simulink model "controlSimulation"  (R2018a)
settings: Solver=VariableStepAuto  StartTime=0.0  StopTime=30  FixedStep=0.01  MaxStep=0.05  RelTol=1e-3  EnableMultiTasking=on
libraries: simulink x1
settings Model: Creator=kk  LastModifiedBy=kk
settings DataIOCC: LimitDataPoints=on  SaveFormat=Array  SaveOutput=off  SignalLogging=off  DSMLogging=off  SaveTime=off
settings OptimizationCC: LifeSpan=inf
settings DebuggingCC: SolverPrmCheckMsg=warning  SFUnexpectedBacktrackingDiag=warning  SFNoUnconditionalDefaultTransitionDiag=warning  SFExecutionAtInitializationDiag=none
settings HardwareCC: ProdBitPerPointer=32  ProdBitPerSizeT=32  ProdBitPerPtrDiffT=32  ProdLargestAtomicFloat=None  ProdIntDivRoundTo=Undefined  ProdEndianess=Unspecified  ProdWordSize=32  ProdHWDeviceType=32-bit Generic
settings ModelReferenceCC: PropagateSignalLabelsOutOfModel=off
settings CodeAppCC: StateflowObjectComments=on
settings GRTTargetCC: TargetLangStandard=C89/C90 (ANSI)  GeneratePreprocessorConditionals=Disable all
settings ConfigComp: CovMetricSettings=dw  CovHtmlReporting=on  CovSaveCumulativeToWorkspaceVar=on  CovSaveSingleToWorkspaceVar=on  CovExternalEMLEnable=off  CovSFcnEnable=off

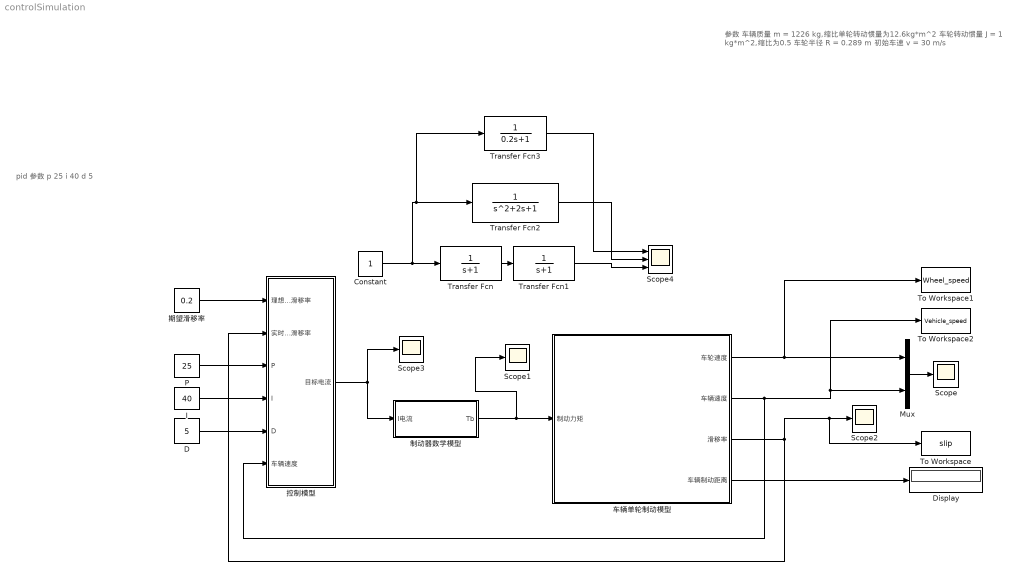
== system controlSimulation ==
  note: pid 参数
      | p 25
      | i 40
      | d 5
  note: 参数
      | 车辆质量 m = 1226 kg,缩比单轮转动惯量为12.6kg*m^2
      | 车轮转动惯量 J = 1 kg*m^2,缩比为0.5
      | 车轮半径 R = 0.289 m
      | 初始车速 v = 30 m/s
  Constant : Constant
  D : Constant  Value=5
  Display : Display
  I : Constant  Value=40
  Mux : Mux  Inputs=2
  P : Constant  Value=25
  Scope{,1..3} (4 alike) : Scope
  Scope4 : Scope  NumInputPorts=3
  To Workspace : ToWorkspace  VariableName=slip  SaveFormat=Timeseries  SampleTime=-1
  To Workspace1 : ToWorkspace  VariableName=Wheel_speed  SaveFormat=Timeseries  SampleTime=-1
  To Workspace2 : ToWorkspace  VariableName=Vehicle_speed  SaveFormat=Timeseries  SampleTime=-1
  Transfer Fcn : TransferFcn  Numerator=1  Denominator=[1 1]
  Transfer Fcn1 : TransferFcn  Numerator=1  Denominator=[1 1]
  Transfer Fcn2 : TransferFcn  Numerator=1
  Transfer Fcn3 : TransferFcn  Numerator=1  Denominator=[0.2 1]
  制动器数学模型 : Subsystem
  控制模型 : Subsystem
  期望滑移率 : Constant  Value=0.2
  车辆单轮制动模型 : Subsystem  mask{v=30, r=0.289, I=0.98/2, m=306.5/2, g=9.8, att=1}
      mask prompts: v "InitialVelocity(v  m/s)"; r "RollingRadius"; I "inertia of a wheel"; m "1/4 Vehicle weight"; g "GravityAcceleration"; att "Attachment condition"
      mask TypeOptions att: 1 | 2 | 3
      mask DialogControl Control2 Prompt: high 1 mediam 2 low 3
  wires:
  期望滑移率/1 -> 控制模型/1(理想滑移率)
  车辆单轮制动模型/3(滑移率) -> To Workspace/1, Scope2/1, 控制模型/2(实时滑移率)
  车辆单轮制动模型/1(车轮速度) -> To Workspace1/1, Mux/1
  Mux/1 -> Scope/1
  P/1 -> 控制模型/3(P)
  I/1 -> 控制模型/4(I)
  D/1 -> 控制模型/5(D)
  车辆单轮制动模型/4(车辆制动距离) -> Display/1
  制动器数学模型/1(Tb) -> Scope1/1, 车辆单轮制动模型/1(制动力矩)
  控制模型/1(目标电流) -> Scope3/1, 制动器数学模型/1(I电流)
  车辆单轮制动模型/2(车辆速度) -> To Workspace2/1, Mux/2, 控制模型/6(车辆速度)
  Constant/1 -> Transfer Fcn3/1, Transfer Fcn2/1, Transfer Fcn/1
  Transfer Fcn/1 -> Transfer Fcn1/1
  Transfer Fcn1/1 -> Scope4/3
  Transfer Fcn2/1 -> Scope4/2
  Transfer Fcn3/1 -> Scope4/1

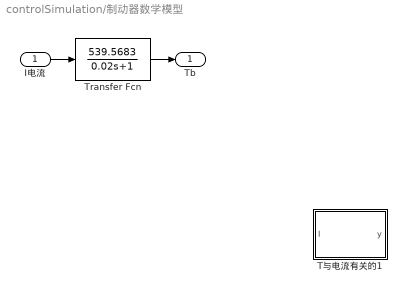
== system controlSimulation/制动器数学模型 ==
  I电流 : Inport
  Transfer Fcn : TransferFcn  Numerator=[539.5683]  Denominator=[0.02 1]
  T与电流有关的1 : MATLAB Function  TreatAsAtomicUnit=on
  Tb : Outport
  wires:
  Transfer Fcn/1 -> Tb/1
  I电流/1 -> Transfer Fcn/1

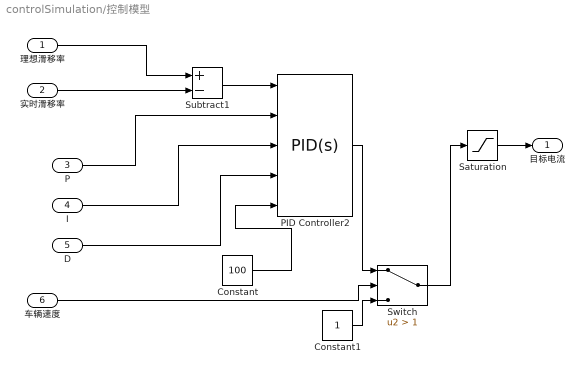
== system controlSimulation/控制模型 ==
  理想滑移率 : Inport
  实时滑移率 : Inport  Port=2
  P : Inport  Port=3
  I : Inport  Port=4
  D : Inport  Port=5
  车辆速度 : Inport  Port=6
  Constant : Constant  Value=100
  Constant1 : Constant
  PID Controller2 : simulink/Continuous/PID Controller  Controller=PID  TimeDomain=Continuous-time  SampleTime=-1  IntegratorMethod=Forward Euler  FilterMethod=Forward Euler  Form=Parallel  UseFilter=on  ControllerParametersSource=external  P=100  I=0  D=0  N=0  InitialConditionSource=internal  InitialConditionForIntegrator=0  InitialConditionForFilter=0  ExternalReset=none  ZeroCross=off  LimitOutput=off  UpperSaturationLimit=3  LowerSaturationLimit=0  LinearizeAsGain=off  AntiWindupMode=none  Kb=1  TrackingMode=off  Kt=1  PParamMin=[]  PParamMax=[]  IParamMin=[]  IParamMax=[]  DParamMin=[]  DParamMax=[]  NParamMin=[]  NParamMax=[]  KbParamMin=[]  KbParamMax=[]  KtParamMin=[]  KtParamMax=[]  POutMin=[]  POutMax=[]  IOutMin=[]  IOutMax=[]  DOutMin=[]  DOutMax=[]  NOutMin=[]  NOutMax=[]  KbOutMin=[]  KbOutMax=[]  KtOutMin=[]  KtOutMax=[]  IntegratorOutMin=[]  IntegratorOutMax=[]  FilterOutMin=[]  FilterOutMax=[]  SumOutMin=[]  SumOutMax=[]  SumI1OutMin=[]  SumI1OutMax=[]  SumI2OutMin=[]  SumI2OutMax=[]  SumI3OutMin=[]  SumI3OutMax=[]  SumDOutMin=[]  SumDOutMax=[]  SaturationOutMin=[]  SaturationOutMax=[]  IntegratorContinuousStateAttributes=''  IntegratorStateMustResolveToSignalObject=off  IntegratorRTWStateStorageClass=Auto  FilterContinuousStateAttributes=''  FilterStateMustResolveToSignalObject=off  FilterRTWStateStorageClass=Auto  DifferentiatorICPrevScaledInput=0  DifferentiatorOutMin=[]  DifferentiatorOutMax=[]  FilterDiffOutCoefMin=[]  FilterDiffOutCoefMax=[]  SumDenOutMin=[]  SumDenOutMax=[]  SumNumOutMin=[]  SumNumOutMax=[]  ReciprocalOutMin=[]  ReciprocalOutMax=[]  DivideOutMin=[]  DivideOutMax=[]  TunerSelectOption=Frequency Response Based
  Saturation : Saturate  UpperLimit=1.2  LowerLimit=0
  Subtract1 : Sum  Inputs=+-
  Switch : Switch  Criteria=u2 > Threshold  Threshold=1
  目标电流 : Outport
  wires:
  Subtract1/1 -> PID Controller2/1
  理想滑移率/1 -> Subtract1/1
  P/1 -> PID Controller2/2
  I/1 -> PID Controller2/3
  D/1 -> PID Controller2/4
  Constant/1 -> PID Controller2/5
  实时滑移率/1 -> Subtract1/2
  车辆速度/1 -> Switch/2
  PID Controller2/1 -> Switch/1
  Constant1/1 -> Switch/3
  Saturation/1 -> 目标电流/1
  Switch/1 -> Saturation/1

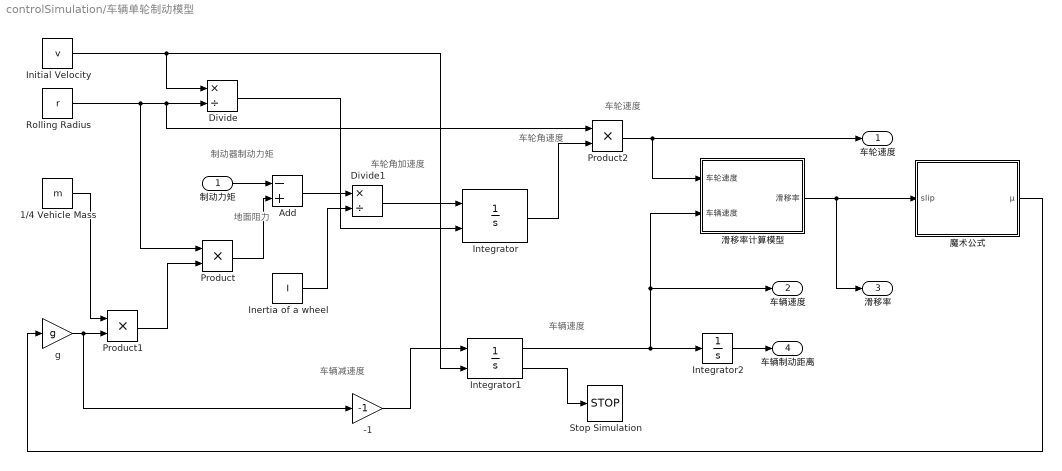
== system controlSimulation/车辆单轮制动模型 ==
  note: 车辆速度
  note: 车辆减速度
  note: 制动器制动力矩
  note: 地面阻力
  note: 车轮角加速度
  note: 车轮角速度
  note: 车轮速度
  制动力矩 : Inport
  -1 : Gain  Gain=-1
  1/4 Vehicle Mass : Constant  Value=m
  Add : Sum  Inputs=-+
  Divide : Product  Inputs=*/
  Divide1 : Product  Inputs=*/
  Inertia of a wheel : Constant  Value=I
  "Initial Velocity " : Constant  Value=v
  Integrator : Integrator  InitialConditionSource=external  InitialCondition=30/0.23  LimitOutput=on  LowerSaturationLimit=0  ZeroCross=off
  Integrator1 : Integrator  InitialConditionSource=external  InitialCondition=30  LimitOutput=on  LowerSaturationLimit=0  ShowSaturationPort=on  ZeroCross=off
  Integrator2 : Integrator
  Product : Product
  Product1 : Product
  Product2 : Product
  "Rolling Radius " : Constant  Value=r
  Stop Simulation : Stop
  g : Gain  Gain=g
  滑移率计算模型 : Subsystem
  魔术公式 : Subsystem
  车轮速度 : Outport
  车辆速度 : Outport  Port=2
  滑移率 : Outport  Port=3
  车辆制动距离 : Outport  Port=4
  wires:
  Product/1 -> Add/2
  Integrator1/2 -> Stop Simulation/1
  Integrator/1 -> Product2/2
  Add/1 -> Divide1/1
  Divide1/1 -> Integrator/1
  Integrator1/1 -> 滑移率计算模型/2(车辆速度), 车辆速度/1, Integrator2/1
  Product2/1 -> 车轮速度/1, 滑移率计算模型/1(车轮速度)
  滑移率计算模型/1(滑移率) -> 魔术公式/1(slip), 滑移率/1
  制动力矩/1 -> Add/1
  "Initial Velocity "/1 -> Integrator1/2, Divide/1
  "Rolling Radius "/1 -> Product2/1, Divide/2, Product/1
  g/1 -> -1/1, Product1/2
  Product1/1 -> Product/2
  魔术公式/1(μ) -> g/1
  -1/1 -> Integrator1/1
  Divide/1 -> Integrator/2
  Integrator2/1 -> 车辆制动距离/1
  1/4 Vehicle Mass/1 -> Product1/1
  Inertia of a wheel/1 -> Divide1/2

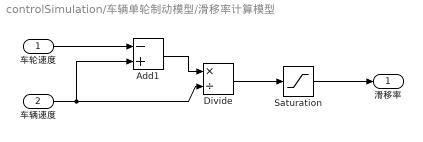
== system controlSimulation/车辆单轮制动模型/滑移率计算模型 ==
  车轮速度 : Inport
  车辆速度 : Inport  Port=2
  Add1 : Sum  Inputs=-+
  Divide : Product  Inputs=*/
  Saturation : Saturate  UpperLimit=1  LowerLimit=0
  滑移率 : Outport
  wires:
  Add1/1 -> Divide/1
  车辆速度/1 -> Add1/2, Divide/2
  Divide/1 -> Saturation/1
  车轮速度/1 -> Add1/1
  Saturation/1 -> 滑移率/1

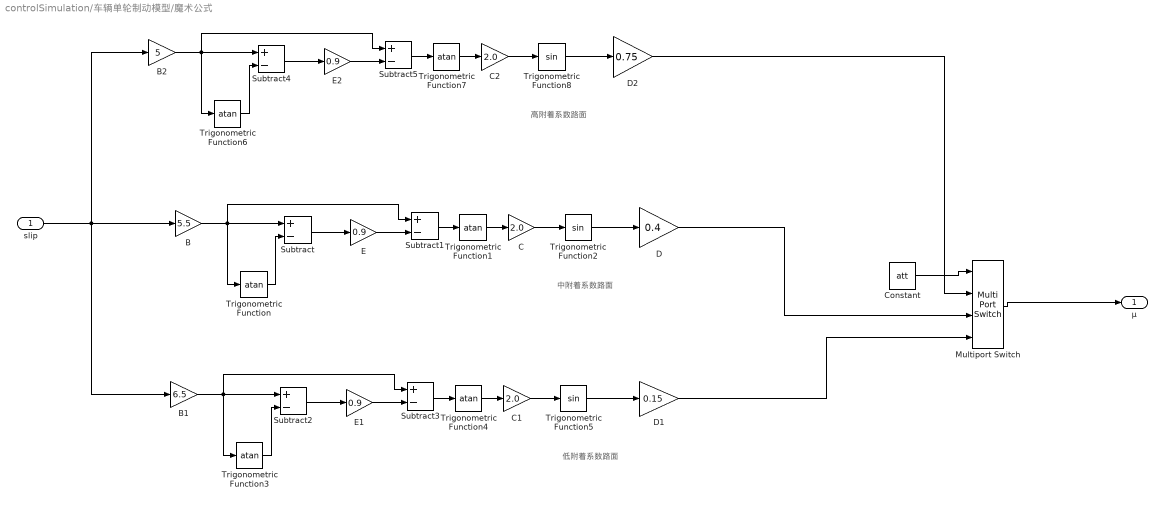
== system controlSimulation/车辆单轮制动模型/魔术公式 ==
  note: 中附着系数路面
  note: 低附着系数路面
  note: 高附着系数路面
  slip : Inport
  B : Gain  Gain=5.5
  B1 : Gain  Gain=6.5
  B2 : Gain  Gain=5
  C : Gain  Gain=2.0
  C1 : Gain  Gain=2.0
  C2 : Gain  Gain=2.0
  Constant : Constant  Value=att
  D : Gain  Gain=0.4
  D1 : Gain  Gain=0.15
  D2 : Gain  Gain=0.75
  E : Gain  Gain=0.9
  E1 : Gain  Gain=0.9
  E2 : Gain  Gain=0.9
  Multiport Switch : MultiPortSwitch
  Subtract{,1..5} (6 alike) : Sum  Inputs=+-
  Trigonometric Function{,1,3..4,6..7} (6 alike) : Trigonometry  Operator=atan
  Trigonometric Function2 : Trigonometry
  Trigonometric Function5 : Trigonometry
  Trigonometric Function8 : Trigonometry
  μ : Outport
  wires:
  C/1 -> Trigonometric Function2/1
  Trigonometric Function/1 -> Subtract/2
  E/1 -> Subtract1/2
  B/1 -> Subtract1/1, Trigonometric Function/1, Subtract/1
  Trigonometric Function1/1 -> C/1
  Trigonometric Function2/1 -> D/1
  Subtract/1 -> E/1
  Subtract1/1 -> Trigonometric Function1/1
  C1/1 -> Trigonometric Function5/1
  Trigonometric Function3/1 -> Subtract2/2
  E1/1 -> Subtract3/2
  B1/1 -> Subtract3/1, Trigonometric Function3/1, Subtract2/1
  Trigonometric Function4/1 -> C1/1
  Trigonometric Function5/1 -> D1/1
  Subtract2/1 -> E1/1
  Subtract3/1 -> Trigonometric Function4/1
  D/1 -> Multiport Switch/3
  D1/1 -> Multiport Switch/4
  D2/1 -> Multiport Switch/2
  Subtract4/1 -> E2/1
  Subtract5/1 -> Trigonometric Function7/1
  E2/1 -> Subtract5/2
  Trigonometric Function8/1 -> D2/1
  B2/1 -> Subtract5/1, Trigonometric Function6/1, Subtract4/1
  slip/1 -> B2/1, B1/1, B/1
  C2/1 -> Trigonometric Function8/1
  Trigonometric Function7/1 -> C2/1
  Trigonometric Function6/1 -> Subtract4/2
  Multiport Switch/1 -> μ/1
  Constant/1 -> Multiport Switch/1

== matlab function controlSimulation/制动器数学模型/T与电流有关的1 ==
  data: I input; y output
function y = fcn(I)
% 参数设置
r1=0.037;r2=0.105;r3=0.139;r4=0.153;
del=0.001;
l1=0.044;l2=0.015;l3=0.008;l4=0.007;
N=1790;%匝数
u1=4*10^-4;%20钢
%u2=4*3.14*10^-7;%不锈钢
u3=3.2*10^-6;%磁流变液
n=3;xiaolv= 1;

% 计算B_I关系
Rm1=(l1+l2)/(pi*u1*(r4^2-r3^2));
Rm2=log((r4+r3)/(r1+r2))/(2*pi*u1*l2);
Rm3=del/(pi*u3*(r2^2-r1^2));

Rm4=l3/(pi*u1*(r2^2-r1^2));
Rm5=l4/(pi*u1*(r2^2-r1^2));

Rm=Rm1+2*Rm2+6*Rm3+3*Rm4+2*Rm5;
S0=pi*(r2^2-r1^2);
k = N/(Rm*S0);
b = k*I*xiaolv;

%计算tau_B
tau= 127.1339*b.^4-318.0875*b.^3+202.0143*b.^2+40.8614*b-0.4536;

%T_tau
y=4/3*pi*n*tau*1000*(r2^3-r1^3);
